simulink model "SM_3_Oc_Vm_Gcm"  (R2021b)
settings: Solver=VariableStepAuto  StartTime=0.0  StopTime=5.2  RelTol=1e-3
settings Model: Creator=sama1402  LastModifiedBy=sama1402

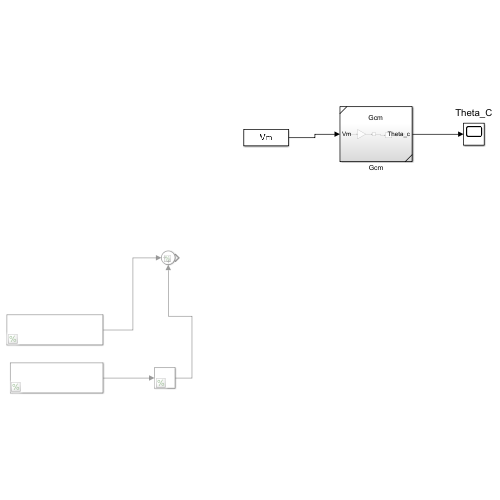
[thumbnail: Simulink's stored preview of the top-level diagram]
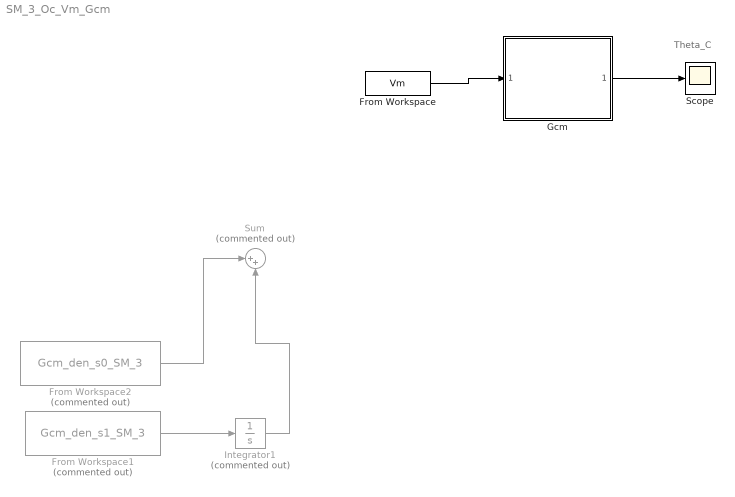
== system SM_3_Oc_Vm_Gcm ==
  note: Theta_C
  From Workspace : FromWorkspace  VariableName=Vm
  From Workspace1 : FromWorkspace  Commented=on  VariableName=Gcm_den_s1_SM_3
  From Workspace2 : FromWorkspace  Commented=on  VariableName=Gcm_den_s0_SM_3
  Gcm : Subsystem  ReferencedSubsystem=Gcm
  Integrator1 : Integrator  Commented=on
  Scope : Scope
  Sum : Sum  Commented=on  Inputs=|++
  wires:
  From Workspace1/1 -> Integrator1/1
  Integrator1/1 -> Sum/2
  From Workspace2/1 -> Sum/1
  From Workspace/1 -> Gcm/1
  Gcm/1 -> Scope/1
